simulink model "all_together_simu_v2"  (R2020b)
settings: Solver=FixedStepDiscrete  StartTime=0.0  StopTime=simTime  RelTol=1e-3
InitFcn:
  | setup
values from neighbouring files (symbols this model uses):
  COLS = 752    [setup.m]    (also in setup_old.m = 640)
  Hh = abs(V(:,1)'*sqrt(S(1,1)))    [setup_old.m]
  Hv = abs(U(:,1)*sqrt(S(1,1)))    [setup_old.m]
undefined symbols (not defined in the file or in its folder): gray, Rec, SDTV
libraries: hdlsllib x52, visionhdlio x7, visionsinks x3, simulink x2, visionconversions x1, visionsources x1
(part 2 of 2)

== system all_together_simu_v2/Gradient Filter/CordicAtan2/Iteration_6/Y_Logic/n_zsign ==
  signof : Inport
  base : Inport  Port=2
  Bit Slice : hdlsllib/Logic and Bit Operations/Bit Slice  lidx=15  ridx=15
      settings: SourceProductBaseCode=SL
  Switch : Switch  Criteria=u2 > Threshold
  Unary Minus : UnaryMinus
  out : Outport
  wires:
  Bit Slice/1 -> Switch/2
  signof/1 -> Bit Slice/1
  base/1 -> Switch/1, Unary Minus/1
  Switch/1 -> out/1
  Unary Minus/1 -> Switch/3

== system all_together_simu_v2/Gradient Filter/CordicAtan2/Iteration_7/X_Logic/zsign ==
  signof : Inport
  base : Inport  Port=2
  Bit Slice : hdlsllib/Logic and Bit Operations/Bit Slice  lidx=15  ridx=15
      settings: SourceProductBaseCode=SL
  Switch : Switch  Criteria=u2 > Threshold
  Unary Minus : UnaryMinus
  out : Outport
  wires:
  signof/1 -> Bit Slice/1
  Bit Slice/1 -> Switch/2
  base/1 -> Switch/3, Unary Minus/1
  Switch/1 -> out/1
  Unary Minus/1 -> Switch/1

== system all_together_simu_v2/Gradient Filter/CordicAtan2/Iteration_7/Y_Logic/n_zsign ==
  signof : Inport
  base : Inport  Port=2
  Bit Slice : hdlsllib/Logic and Bit Operations/Bit Slice  lidx=15  ridx=15
      settings: SourceProductBaseCode=SL
  Switch : Switch  Criteria=u2 > Threshold
  Unary Minus : UnaryMinus
  out : Outport
  wires:
  Bit Slice/1 -> Switch/2
  signof/1 -> Bit Slice/1
  base/1 -> Switch/1, Unary Minus/1
  Switch/1 -> out/1
  Unary Minus/1 -> Switch/3

== system all_together_simu_v2/Gradient Filter/CordicAtan2/Iteration_8/X_Logic/zsign ==
  signof : Inport
  base : Inport  Port=2
  Bit Slice : hdlsllib/Logic and Bit Operations/Bit Slice  lidx=15  ridx=15
      settings: SourceProductBaseCode=SL
  Switch : Switch  Criteria=u2 > Threshold
  Unary Minus : UnaryMinus
  out : Outport
  wires:
  signof/1 -> Bit Slice/1
  Bit Slice/1 -> Switch/2
  base/1 -> Switch/3, Unary Minus/1
  Switch/1 -> out/1
  Unary Minus/1 -> Switch/1

== system all_together_simu_v2/Gradient Filter/CordicAtan2/Iteration_8/Y_Logic/n_zsign ==
  signof : Inport
  base : Inport  Port=2
  Bit Slice : hdlsllib/Logic and Bit Operations/Bit Slice  lidx=15  ridx=15
      settings: SourceProductBaseCode=SL
  Switch : Switch  Criteria=u2 > Threshold
  Unary Minus : UnaryMinus
  out : Outport
  wires:
  Bit Slice/1 -> Switch/2
  signof/1 -> Bit Slice/1
  base/1 -> Switch/1, Unary Minus/1
  Switch/1 -> out/1
  Unary Minus/1 -> Switch/3

== system all_together_simu_v2/Gradient Filter/CordicAtan2/Iteration_9/X_Logic/zsign ==
  signof : Inport
  base : Inport  Port=2
  Bit Slice : hdlsllib/Logic and Bit Operations/Bit Slice  lidx=15  ridx=15
      settings: SourceProductBaseCode=SL
  Switch : Switch  Criteria=u2 > Threshold
  Unary Minus : UnaryMinus
  out : Outport
  wires:
  signof/1 -> Bit Slice/1
  Bit Slice/1 -> Switch/2
  base/1 -> Switch/3, Unary Minus/1
  Switch/1 -> out/1
  Unary Minus/1 -> Switch/1

== system all_together_simu_v2/Gradient Filter/CordicAtan2/Iteration_9/Y_Logic/n_zsign ==
  signof : Inport
  base : Inport  Port=2
  Bit Slice : hdlsllib/Logic and Bit Operations/Bit Slice  lidx=15  ridx=15
      settings: SourceProductBaseCode=SL
  Switch : Switch  Criteria=u2 > Threshold
  Unary Minus : UnaryMinus
  out : Outport
  wires:
  Bit Slice/1 -> Switch/2
  signof/1 -> Bit Slice/1
  base/1 -> Switch/1, Unary Minus/1
  Switch/1 -> out/1
  Unary Minus/1 -> Switch/3

== system all_together_simu_v2/Gradient Filter/Ix//Iy Filters/Ix Filter/Filter/Row Filter2 ==
  data_in : Inport
  Delay : Delay  DelayLength=4
  Symmetry : Subsystem
  data_out : Outport
  wires:
  Symmetry/1(data_out) -> Delay/1
  data_in/1 -> Symmetry/1(data_in)
  Delay/1 -> data_out/1

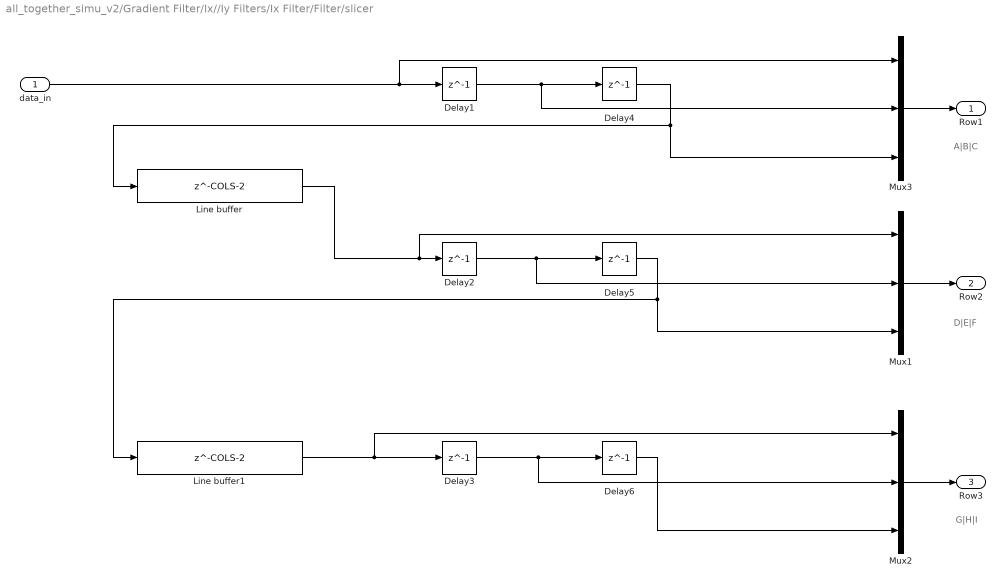
== system all_together_simu_v2/Gradient Filter/Ix//Iy Filters/Ix Filter/Filter/slicer ==
  note: A|B|C
  note: D|E|F
  note: G|H|I
  data_in : Inport
  Delay{1..6} (6 alike) : Delay  DelayLength=1  InitialCondition=0
  Line buffer : Delay  DelayLength=COLS-2  InitialCondition=0
  Line buffer1 : Delay  DelayLength=COLS-2  InitialCondition=0
  Mux1 : Mux  Inputs=3
  Mux2 : Mux  Inputs=3
  Mux3 : Mux  Inputs=3
  Row1 : Outport  VectorParamsAs1DForOutWhenUnconnected=off
  Row2 : Outport  Port=2  VectorParamsAs1DForOutWhenUnconnected=off
  Row3 : Outport  Port=3  VectorParamsAs1DForOutWhenUnconnected=off
  wires:
  Delay4/1 -> Mux3/3, Line buffer/1
  data_in/1 -> Mux3/1, Delay1/1
  Delay1/1 -> Mux3/2, Delay4/1
  Delay3/1 -> Mux2/2, Delay6/1
  Delay5/1 -> Mux1/3, Line buffer1/1
  Delay6/1 -> Mux2/3
  Line buffer/1 -> Mux1/1, Delay2/1
  Line buffer1/1 -> Mux2/1, Delay3/1
  Delay2/1 -> Mux1/2, Delay5/1
  Mux1/1 -> Row2/1
  Mux2/1 -> Row3/1
  Mux3/1 -> Row1/1

== system all_together_simu_v2/Gradient Filter/Ix//Iy Filters/Iy Filter/Filter/Row Filter1 ==
  data_in : Inport
  Delay : Delay
  Symmetry : Subsystem
  data_out : Outport
  wires:
  Symmetry/1(data_out) -> Delay/1
  data_in/1 -> Symmetry/1(data_in)
  Delay/1 -> data_out/1

== system all_together_simu_v2/Gradient Filter/Ix//Iy Filters/Iy Filter/Filter/Row Filter3 ==
  data_in : Inport
  Delay : Delay
  Symmetry : Subsystem
  data_out : Outport
  wires:
  Symmetry/1(data_out) -> Delay/1
  data_in/1 -> Symmetry/1(data_in)
  Delay/1 -> data_out/1

== system all_together_simu_v2/Gradient Filter/Ix//Iy Filters/Iy Filter/Filter/Verticle Filter ==
  data_in : Inport
  Delay2 : Delay
  Symmetry : Subsystem
  data_out : Outport
  wires:
  Delay2/1 -> data_out/1
  data_in/1 -> Symmetry/1(data_in)
  Symmetry/1(data_out) -> Delay2/1

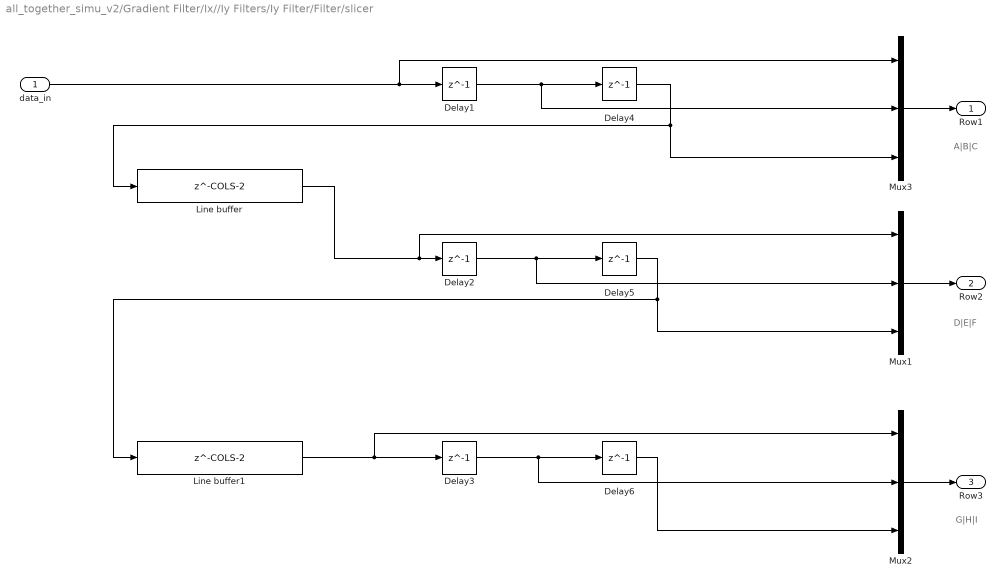
== system all_together_simu_v2/Gradient Filter/Ix//Iy Filters/Iy Filter/Filter/slicer ==
  note: A|B|C
  note: D|E|F
  note: G|H|I
  data_in : Inport
  Delay{1..6} (6 alike) : Delay  DelayLength=1  InitialCondition=0
  Line buffer : Delay  DelayLength=COLS-2  InitialCondition=0
  Line buffer1 : Delay  DelayLength=COLS-2  InitialCondition=0
  Mux1 : Mux  Inputs=3
  Mux2 : Mux  Inputs=3
  Mux3 : Mux  Inputs=3
  Row1 : Outport  VectorParamsAs1DForOutWhenUnconnected=off
  Row2 : Outport  Port=2  VectorParamsAs1DForOutWhenUnconnected=off
  Row3 : Outport  Port=3  VectorParamsAs1DForOutWhenUnconnected=off
  wires:
  Delay4/1 -> Mux3/3, Line buffer/1
  data_in/1 -> Mux3/1, Delay1/1
  Delay1/1 -> Mux3/2, Delay4/1
  Delay3/1 -> Mux2/2, Delay6/1
  Delay5/1 -> Mux1/3, Line buffer1/1
  Delay6/1 -> Mux2/3
  Line buffer/1 -> Mux1/1, Delay2/1
  Line buffer1/1 -> Mux2/1, Delay3/1
  Delay2/1 -> Mux1/2, Delay5/1
  Mux1/1 -> Row2/1
  Mux2/1 -> Row3/1
  Mux3/1 -> Row1/1

== system all_together_simu_v2/Gradient Filter/Ix//Iy Filters/Ix Filter/Filter/Row Filter2/Symmetry ==
  data_in : Inport
  Demux : Demux  Outputs=3
  Mux : Mux  Inputs=1
  Sum3 : Sum  Inputs=|+-
  Terminator : Terminator
  data_out : Outport
  wires:
  Sum3/1 -> Mux/1
  data_in/1 -> Demux/1
  Demux/2 -> Terminator/1
  Demux/3 -> Sum3/2
  Demux/1 -> Sum3/1
  Mux/1 -> data_out/1

== system all_together_simu_v2/Gradient Filter/Ix//Iy Filters/Iy Filter/Filter/Row Filter1/Symmetry ==
  data_in : Inport
  Demux : Demux  Outputs=3
  Mux : Mux  Inputs=1
  Terminator : Terminator
  Terminator1 : Terminator
  data_out : Outport
  wires:
  data_in/1 -> Demux/1
  Demux/2 -> Mux/1
  Mux/1 -> data_out/1
  Demux/1 -> Terminator/1
  Demux/3 -> Terminator1/1

== system all_together_simu_v2/Gradient Filter/Ix//Iy Filters/Iy Filter/Filter/Row Filter3/Symmetry ==
  data_in : Inport
  Demux : Demux  Outputs=3
  Mux : Mux  Inputs=1
  Terminator : Terminator
  Terminator1 : Terminator
  data_out : Outport
  wires:
  data_in/1 -> Demux/1
  Demux/2 -> Mux/1
  Mux/1 -> data_out/1
  Demux/1 -> Terminator/1
  Demux/3 -> Terminator1/1

== system all_together_simu_v2/Gradient Filter/Ix//Iy Filters/Iy Filter/Filter/Verticle Filter/Symmetry ==
  data_in : Inport
  Demux : Demux  Outputs=3
  Mux : Mux  Inputs=1
  Sum : Sum  Inputs=|+-
  Terminator : Terminator
  data_out : Outport
  wires:
  data_in/1 -> Demux/1
  Demux/2 -> Terminator/1
  Mux/1 -> data_out/1
  Demux/1 -> Sum/1
  Demux/3 -> Sum/2
  Sum/1 -> Mux/1
